simulink model "state_estimator"  (R2018b)
settings: Solver=VariableStepAuto  StartTime=0.0  StopTime=inf  RelTol=1e-3
libraries: simulink_extras x9, sharedTrackingLibrary x2, Solver_SF x1
settings Model: Creator=tusen  LastModifiedBy=tusen

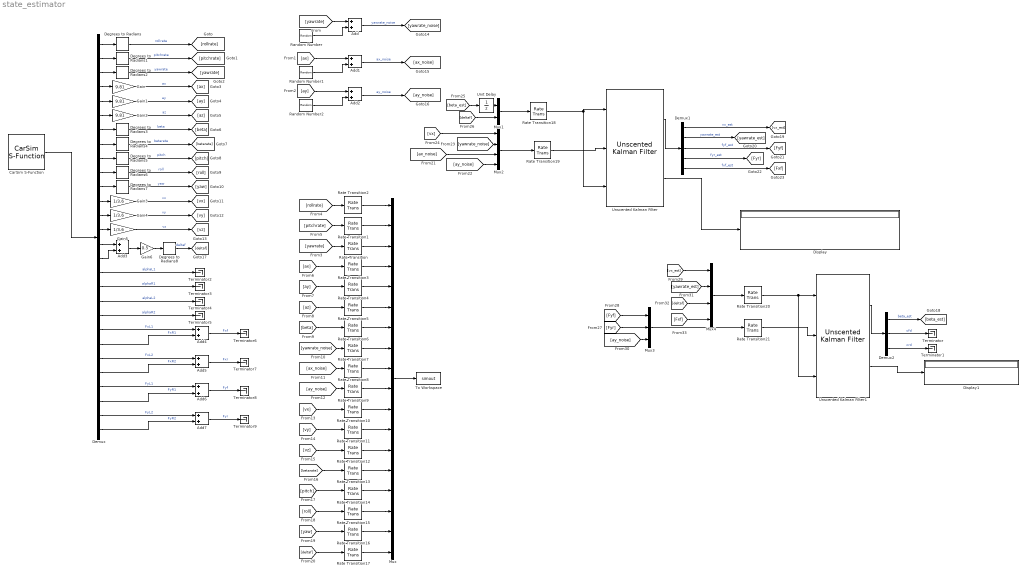
== system state_estimator ==
  Add{,1..7} (8 alike) : Sum
  CarSim S-Function : Solver_SF/CarSim S-Function  Priority=1  SIMFILE=simfile.sim  Run_RTs=off  vs_state_ind=Run  StopMode_ind=Vehicle Model
  Degrees to Radians{,1..8} (9 alike) : simulink_extras/Transformations/Degrees to Radians
  Demux : Demux  Outputs=28
  Demux1 : Demux  Outputs=5
  Demux2 : Demux  Outputs=3
  Display : Display
  Display1 : Display
  Gain : Gain  Gain=9.81
  Gain1 : Gain  Gain=9.81
  Gain2 : Gain  Gain=9.81
  Gain3 : Gain  Gain=1/3.6
  Gain4 : Gain  Gain=1/3.6
  Gain5 : Gain  Gain=1/3.6
  Gain6 : Gain  Gain=0.5
  Mux : Mux  Inputs=18
  Mux1 : Mux  Inputs=2
  Mux2 : Mux
  Mux3 : Mux  Inputs=3
  Mux4 : Mux
  Random Number : RandomNumber  Variance=0.2  SampleTime=0.01
  Random Number1 : RandomNumber  Variance=0.2  SampleTime=0.01
  Random Number2 : RandomNumber  Variance=0.2  SampleTime=0.01
  Rate Transition{,1..21} (22 alike) : RateTransition  OutPortSampleTime=0.01
  Terminator{,1..9} (10 alike) : Terminator
  To Workspace : ToWorkspace  VariableName=simout  SaveFormat=Structure With Time  SampleTime=-1
  Unit Delay : UnitDelay  SampleTime=-1
  Unscented Kalman Filter : sharedTrackingLibrary/Unscented Kalman Filter  StateTransitionFcn=StateA  HasAdditiveProcessNoise=Additive  ProcessNoise=[1e-5,0,0,0,0;0,1e-6,0,0,0;0,0,1e5,0,0;0,0,0,1e3,0;0,0,0,0,1e3]  HasTimeVaryingProcessNoise=off  HasStateTransitionFcnExtraArgument=1  InitialState=zeros(5,1)  InitialStateCovariance=eye(5)  Alpha=1e-3  Beta=2  Kappa=0  MeasurementFcn1=MeasureA  HasMeasurementEnablePort1=off  HasAdditiveMeasurementNoise1=Additive  MeasurementNoise1=[1e-4,0,0,0;0,0.2,0,0;0,0,0.2,0;0,0,0,0.2]  HasTimeVaryingMeasurementNoise1=off  HasMeasurementFcnExtraArgument1=1  MeasurementFcn2=myMeasurementFcn  HasMeasurementEnablePort2=off  HasAdditiveMeasurementNoise2=Additive  MeasurementNoise2=1  HasTimeVaryingMeasurementNoise2=off  HasMeasurementFcnExtraArgument2=0  MeasurementFcn3=myMeasurementFcn  HasMeasurementEnablePort3=off  HasAdditiveMeasurementNoise3=Additive  MeasurementNoise3=1  HasTimeVaryingMeasurementNoise3=off  HasMeasurementFcnExtraArgument3=0  MeasurementFcn4=myMeasurementFcn  HasMeasurementEnablePort4=off  HasAdditiveMeasurementNoise4=Additive  MeasurementNoise4=1  HasTimeVaryingMeasurementNoise4=off  HasMeasurementFcnExtraArgument4=0  MeasurementFcn5=myMeasurementFcn  HasMeasurementEnablePort5=off  HasAdditiveMeasurementNoise5=Additive  MeasurementNoise5=1  HasTimeVaryingMeasurementNoise5=off  HasMeasurementFcnExtraArgument5=0  EnableMultirate=off  StateTransitionFcnSampleTime=1  MeasurementFcn1SampleTime=1  MeasurementFcn2SampleTime=1  MeasurementFcn3SampleTime=1  MeasurementFcn4SampleTime=1  MeasurementFcn5SampleTime=1  UseCurrentEstimator=on  OutputStateCovariance=on  DataType=double  SampleTime=0.01  NumberOfMeasurements=1
      settings: SourceProductName=Control System Toolbox  SourceProductBaseCode=CT
  Unscented Kalman Filter1 : sharedTrackingLibrary/Unscented Kalman Filter  StateTransitionFcn=StateB  HasAdditiveProcessNoise=Additive  ProcessNoise=[1e-3,0,0;0,1e-10,0;0,0,1e-10;]  HasTimeVaryingProcessNoise=off  HasStateTransitionFcnExtraArgument=1  InitialState=zeros(3,1)  InitialStateCovariance=eye(3)  Alpha=1e-3  Beta=2  Kappa=0  MeasurementFcn1=MeasureB  HasMeasurementEnablePort1=off  HasAdditiveMeasurementNoise1=Additive  MeasurementNoise1=[1e3,0,0;0,1e3,0;0,0,0.02;]  HasTimeVaryingMeasurementNoise1=off  HasMeasurementFcnExtraArgument1=1  MeasurementFcn2=myMeasurementFcn  HasMeasurementEnablePort2=off  HasAdditiveMeasurementNoise2=Additive  MeasurementNoise2=1  HasTimeVaryingMeasurementNoise2=off  HasMeasurementFcnExtraArgument2=0  MeasurementFcn3=myMeasurementFcn  HasMeasurementEnablePort3=off  HasAdditiveMeasurementNoise3=Additive  MeasurementNoise3=1  HasTimeVaryingMeasurementNoise3=off  HasMeasurementFcnExtraArgument3=0  MeasurementFcn4=myMeasurementFcn  HasMeasurementEnablePort4=off  HasAdditiveMeasurementNoise4=Additive  MeasurementNoise4=1  HasTimeVaryingMeasurementNoise4=off  HasMeasurementFcnExtraArgument4=0  MeasurementFcn5=myMeasurementFcn  HasMeasurementEnablePort5=off  HasAdditiveMeasurementNoise5=Additive  MeasurementNoise5=1  HasTimeVaryingMeasurementNoise5=off  HasMeasurementFcnExtraArgument5=0  EnableMultirate=off  StateTransitionFcnSampleTime=1  MeasurementFcn1SampleTime=1  MeasurementFcn2SampleTime=1  MeasurementFcn3SampleTime=1  MeasurementFcn4SampleTime=1  MeasurementFcn5SampleTime=1  UseCurrentEstimator=on  OutputStateCovariance=on  DataType=double  SampleTime=0.01  NumberOfMeasurements=1
      settings: SourceProductName=Control System Toolbox  SourceProductBaseCode=CT
  wires:
  CarSim S-Function/1 -> Demux/1
  Demux/1 -> Degrees to Radians/1
  Demux/2 -> Degrees to Radians1/1
  Demux/3 -> Degrees to Radians2/1
  Demux/4 -> Gain/1
  Demux/5 -> Gain1/1
  Demux/6 -> Gain2/1
  Demux/7 -> Degrees to Radians3/1
  Demux/8 -> Degrees to Radians4/1
  Demux/9 -> Degrees to Radians5/1
  Demux/10 -> Degrees to Radians6/1
  Demux/11 -> Degrees to Radians7/1
  Demux/12 -> Gain3/1
  Demux/13 -> Gain4/1
  Demux/14 -> Gain5/1
  Degrees to Radians/1 -> [rollrate]  "rollrate"
  Degrees to Radians1/1 -> [pitchrate]  "pitchrate"
  Degrees to Radians2/1 -> [yawrate]  "yawrate"
  Degrees to Radians3/1 -> [beta]  "beta"
  Degrees to Radians4/1 -> [betarate]  "betarate"
  Degrees to Radians5/1 -> [pitch]  "pitch"
  Degrees to Radians6/1 -> [roll]  "roll"
  Degrees to Radians7/1 -> [yaw]  "yaw"
  Gain/1 -> [ax]  "ax"
  Gain1/1 -> [ay]  "ay"
  Gain2/1 -> [az]  "az"
  Gain3/1 -> [vx]  "vx"
  Gain4/1 -> [vy]  "vy"
  Gain5/1 -> [vz]  "vz"
  [yawrate] -> Add/1
  Random Number/1 -> Add/2
  Add/1 -> [yawrate_noise]  "yawrate_noise"
  Random Number1/1 -> Add1/2
  [ax] -> Add1/1
  Random Number2/1 -> Add2/2
  [ay] -> Add2/1
  Add1/1 -> [ax_noise]  "ax_noise"
  Add2/1 -> [ay_noise]  "ay_noise"
  [yawrate] -> Rate Transition/1
  [pitchrate] -> Rate Transition1/1
  [rollrate] -> Rate Transition2/1
  [ax] -> Rate Transition3/1
  [ay] -> Rate Transition4/1
  [az] -> Rate Transition5/1
  [beta] -> Rate Transition6/1
  [yawrate_noise] -> Rate Transition7/1
  [ax_noise] -> Rate Transition8/1
  [ay_noise] -> Rate Transition9/1
  [vx] -> Rate Transition10/1
  [vy] -> Rate Transition11/1
  [vz] -> Rate Transition12/1
  [betarate] -> Rate Transition13/1
  [pitch] -> Rate Transition14/1
  [roll] -> Rate Transition15/1
  [yaw] -> Rate Transition16/1
  Rate Transition2/1 -> Mux/1
  Rate Transition1/1 -> Mux/2
  Rate Transition/1 -> Mux/3
  Rate Transition3/1 -> Mux/4
  Rate Transition4/1 -> Mux/5
  Rate Transition5/1 -> Mux/6
  Rate Transition6/1 -> Mux/7
  Rate Transition7/1 -> Mux/8
  Rate Transition8/1 -> Mux/9
  Rate Transition9/1 -> Mux/10
  Rate Transition10/1 -> Mux/11
  Rate Transition11/1 -> Mux/12
  Rate Transition12/1 -> Mux/13
  Rate Transition13/1 -> Mux/14
  Rate Transition14/1 -> Mux/15
  Rate Transition15/1 -> Mux/16
  Rate Transition16/1 -> Mux/17
  Mux/1 -> To Workspace/1
  Demux/15 -> Add3/1
  Demux/16 -> Add3/2
  Add3/1 -> Gain6/1
  Degrees to Radians8/1 -> [deltaf]  "deltaf"
  Rate Transition17/1 -> Mux/18
  [deltaf] -> Rate Transition17/1
  Gain6/1 -> Degrees to Radians8/1
  Mux1/1 -> Rate Transition18/1
  Mux2/1 -> Rate Transition19/1
  [vx] -> Mux2/1
  [yawrate_noise] -> Mux2/2
  [ay_noise] -> Mux2/4
  [ax_noise] -> Mux2/3
  [deltaf] -> Mux1/2
  Unscented Kalman Filter/1 -> Demux1/1
  Unscented Kalman Filter1/1 -> Demux2/1
  Demux2/1 -> [beta_est]  "beta_est"
  Demux2/2 -> Terminator/1  "cfd"
  Demux2/3 -> Terminator1/1  "crd"
  Demux1/1 -> [vx_est]  "vx_est"
  Demux1/2 -> [yawrate_est]  "yawrate_est"
  Demux1/3 -> [Fyf]  "fyf_est"
  Demux1/4 -> [Fyr]  "fyr_est"
  Demux1/5 -> [Fxf]  "fxf_est"
  [ay_noise] -> Mux3/3
  [Fyr] -> Mux3/2
  [Fyf] -> Mux3/1
  Mux3/1 -> Rate Transition21/1
  [vx_est] -> Mux4/1
  [yawrate_est] -> Mux4/2
  [deltaf] -> Mux4/3
  Mux4/1 -> Rate Transition20/1
  [Fxf] -> Mux4/4
  Rate Transition18/1 -> Unscented Kalman Filter/1, Unscented Kalman Filter/3
  Rate Transition19/1 -> Unscented Kalman Filter/2
  Rate Transition20/1 -> Unscented Kalman Filter1/3, Unscented Kalman Filter1/1
  Rate Transition21/1 -> Unscented Kalman Filter1/2
  [beta_est] -> Unit Delay/1
  Unit Delay/1 -> Mux1/1
  Demux/17 -> Terminator2/1  "alphaL1"
  Demux/18 -> Terminator3/1  "alphaR1"
  Demux/19 -> Terminator4/1  "alphaL2"
  Demux/20 -> Terminator5/1  "alphaR2"
  Demux/21 -> Add4/1  "FxL1"
  Demux/22 -> Add4/2  "FxR1"
  Demux/23 -> Add5/1  "FxL2"
  Demux/24 -> Add5/2  "FxR2"
  Demux/25 -> Add6/1  "FyL1"
  Demux/26 -> Add6/2  "FyR1"
  Demux/27 -> Add7/1  "FyL2"
  Demux/28 -> Add7/2  "FyR2"
  Add4/1 -> Terminator6/1  "Fxf"
  Add5/1 -> Terminator7/1  "Fxr"
  Add6/1 -> Terminator8/1  "Fyf"
  Add7/1 -> Terminator9/1  "Fyr"
  Unscented Kalman Filter/2 -> Display/1
  Unscented Kalman Filter1/2 -> Display1/1
